simulink model "BLDC"  (R2023b)
settings: Solver=VariableStepAuto  StartTime=0.0  StopTime=0.25  RelTol=1e-3
libraries: simulink x6, spsPermanentMagnetSynchronousMachineLib x1, spsControlledVoltageSourceLib x1, slpidlib x1, spsUniversalBridgeLib x1, spsVoltageMeasurementLib x1, spspowerguiLib x1
settings Model: Creator=Akaashdeep B  LastModifiedBy=Akaashdeep B

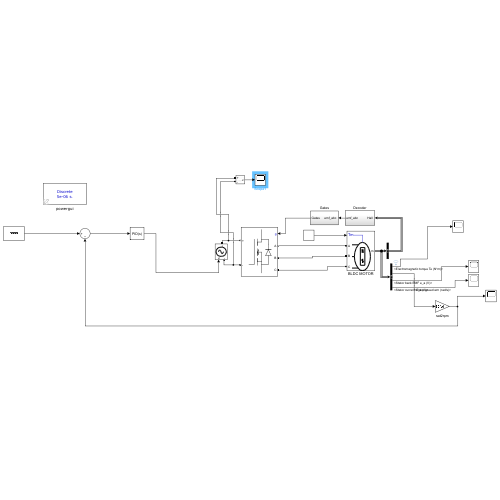
[thumbnail: Simulink's stored preview of the top-level diagram]
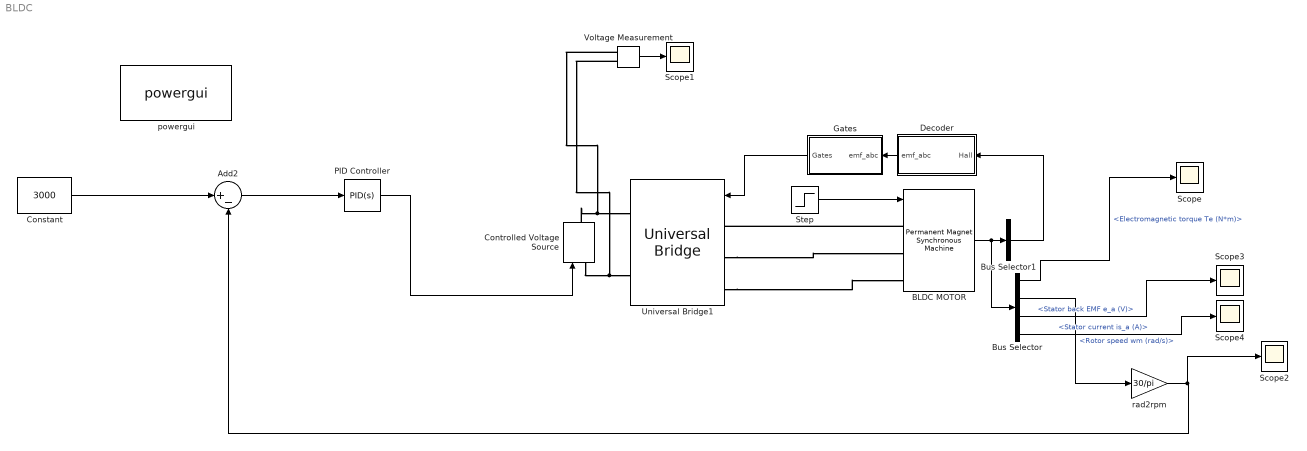
== system BLDC ==
  Add2 : Sum  Inputs=|+-
  BLDC MOTOR : spsPermanentMagnetSynchronousMachineLib/Permanent Magnet Synchronous Machine  NbPhases=3  FluxDistribution=Trapezoidal  RotorType=Round  MechanicalLoad=Torque Tm  PresetModel=No  ShowDetailedParameters=on  MeasurementBus=off  Resistance=2.8750  Inductance=8.5e-3  dqInductances=[8.5e-3, 8.5e-3]  La=0.000835  MachineConstant=Torque Constant (N.m / A_peak)  Flux=0.175  VoltageCst=146.6077  TorqueCst=1.4  Flat=120  Mechanical="[ 0.8e-3, 1e-3,  4 ]"  PolePairs=4  InitialConditions=[0,0, 0,0]  InitialConditions5ph=[0 0 0 0 0 0]  RefAngle=90 degrees behind phase A axis (modified Park)  IterativeDiscreteModel=Trapezoidal non iterative  TsBlock=-1  TsPowergui=0
  Bus Selector : BusSelector  OutputSignals=Electromagnetic torque Te (N*m),Rotor speed wm (rad/s),Stator back EMF e_a (V),Stator current is_a (A)
  Bus Selector1 : BusSelector  OutputSignals=Hall effect signal h_a,Hall effect signal h_b,Hall effect signal h_c  OutputAsBus=on
  Constant : Constant  Value=3000
  Controlled Voltage Source : spsControlledVoltageSourceLib/Controlled Voltage Source  Initialize=on  Source_Type=DC  Amplitude=0  Phase=0  Frequency=50  Measurements=None
  Decoder : Subsystem
  Gates : Subsystem
  PID Controller : slpidlib/PID Controller  Controller=PID  Form=Parallel  TimeDomain=Continuous-time  UseExternalTs=off  SampleTime=-1  IntegratorMethod=Forward Euler  FilterMethod=Forward Euler  ControllerParametersSource=internal  P=0.01035  I=12.777  UseKiTs=off  D=12.564  N=0  UseFilter=on  TunerSelectOption=Transfer Function Based (PID Tuner App)  InitialConditionSource=internal  InitialConditionForIntegrator=0  InitialConditionForFilter=0  DifferentiatorICPrevScaledInput=0  ExternalReset=none  TrackingMode=off  Kt=1  LimitOutput=off  SatLimitsSource=internal  UpperSaturationLimit=inf  LowerSaturationLimit=-inf  LinearizeAsGain=on  AntiWindupMode=none  Kb=1  LimitIntegrator=off  UpperIntegratorSaturationLimit=inf  LowerIntegratorSaturationLimit=-inf  POutMin=[]  POutMax=[]  IOutMin=[]  IOutMax=[]  DOutMin=[]  DOutMax=[]  NOutMin=[]  NOutMax=[]  SumOutMin=[]  SumOutMax=[]  SaturationOutMin=[]  SaturationOutMax=[]  PParamMin=[]  PParamMax=[]  IParamMin=[]  IParamMax=[]  DParamMin=[]  DParamMax=[]  NParamMin=[]  NParamMax=[]  KbParamMin=[]  KbParamMax=[]  KtParamMin=[]  KtParamMax=[]  KbOutMin=[]  KbOutMax=[]  KtOutMin=[]  KtOutMax=[]  IntegratorOutMin=[]  IntegratorOutMax=[]  FilterOutMin=[]  FilterOutMax=[]  SumI1OutMin=[]  SumI1OutMax=[]  SumI2OutMin=[]  SumI2OutMax=[]  SumI3OutMin=[]  SumI3OutMax=[]  SumI4OutMin=[]  SumI4OutMax=[]  SumDOutMin=[]  SumDOutMax=[]  DifferentiatorOutMin=[]  DifferentiatorOutMax=[]  FilterDiffOutCoefMin=[]  FilterDiffOutCoefMax=[]  ReciprocalOutMin=[]  ReciprocalOutMax=[]  SumDenOutMin=[]  SumDenOutMax=[]  SumNumOutMin=[]  SumNumOutMax=[]  DivideOutMin=[]  DivideOutMax=[]  UdiffTsProdOutMin=[]  UdiffTsProdOutMax=[]  NTsProdOutMin=[]  NTsProdOutMax=[]  UintegralTsProdOutMin=[]  UintegralTsProdOutMax=[]  UngainTsProdOutMin=[]  UngainTsProdOutMax=[]  ClampingZeroOutDataTypeStr=Inherit: Inherit via back propagation  ClampingZeroOutMin=[]  ClampingZeroOutMax=[]  FilterDenConstantOutDataTypeStr=Inherit: Inherit via back propagation  FilterDenConstantOutMin=[]  FilterDenConstantOutMax=[]  PCopyOutDataTypeStr=Inherit: Inherit via back propagation  PCopyOutMin=[]  PCopyOutMax=[]  NCopyOutDataTypeStr=Inherit: Inherit via back propagation  NCopyOutMin=[]  NCopyOutMax=[]  IntegratorContinuousStateAttributes=''  IntegratorStateMustResolveToSignalObject=off  IntegratorRTWStateStorageClass=Auto  FilterContinuousStateAttributes=''  FilterStateMustResolveToSignalObject=off  FilterRTWStateStorageClass=Auto  ParallelPVariant=InternalParameters  IdealPVariant=Disabled  IVariant=InternalParameters  DVariant=InternalParameters  IntegratorVariant=Continuous  SatVariant=Disabled  AWVariant=Passthrough  PCopyVariant=Disabled  TRVariant=Disabled  FdbkBlocksVariant=Forward  IdealPFdbkVariant=Disabled  SatFdbkVariant=Disabled  DerivativeFilterVariant=ContFilter  NVariant=InternalParameters  NCopyVariant=Disabled  FilterICVariant=InternalICsFilter  IntegratorICVariant=InternalICs  ExternalResetVariant=Disabled  TRSumVariant=Passthrough  SumFdbkVariant=Disabled  SumVariant=Sum_PID  TsampFilterVariant=InternalTs  TsampNgainVariant=Passthrough  TsampIntegralVariant=Disabled_SignalSpec  ExternalSaturationOutDataTypeStr=Inherit: Same as second input
  Scope{,1..4} (5 alike) : Scope
  Step : Step  Time=0.1  SampleTime=0
  Universal Bridge1 : spsUniversalBridgeLib/Universal Bridge  Arms=3  SnubberResistance=5000  SnubberCapacitance=1e-6  Device=MOSFET / Diodes  Ron=1e-3  Lon=0  ForwardVoltages="[  0  0  ]"  ForwardVoltage=0  GTOparameters=[ 10e-6 , 20e-6 ]  IGBTparameters=[ 1e-6 , 2e-6 ]  Measurements=None  Measurements_2=None  converterType=Rectifier
  Voltage Measurement : spsVoltageMeasurementLib/Voltage Measurement  PhasorSimulation=off  OutputType=Complex  PSBequivalent=0
  powergui : spspowerguiLib/powergui  SimulationMode=Discrete  SampleTime=5e-6  frequency=60  Iterations=50  frequencyindice=0  Pbase=100e6  ErrMax=1e-4  UnitsV=kV  UnitsW=MW  buscounter=0  FunctionMessages=off  echomessages=off  EnableUseOfTLC=off  CurrentSourceSwitches=off  DisableSnubberDevices=off  DisableRonSwitches=off  DisableVfSwitches=off  DisplayEquations=off  AutomaticDiscreteSolvers=off  SolverType=Tustin  Interpol=off  ExternalGateDelay=off  methode=off  Ts=0  x0status=blocks  SPID=off  SwTol=0  HookPort=off  NonlinearTolerance=1e-4  nMaxIteration=100  ContinueOnMaxIteration=off  RestoreLinks=warning  ResistiveCurrentMeasurement=off  Frange=[0:2:500]  Ylog=off  Xlog=on  ShowGrid=off  save=off  variable=ZData  structure=ScopeData7  ZoomFFT=off  StartTime=0.24  cycles=1  DisplayStyle=1  fundamental=50  FreqAxis=on  MaxFrequency=1000  frequencyindicesteady=1  RmsSteady=1  display=off
  rad2rpm : Gain  Gain=30/pi
  wires:
  PID Controller/1 -> Controlled Voltage Source/1
  Bus Selector/1 -> Scope/1  "<Electromagnetic torque Te (N*m)>"
  Gates/1(Gates) -> Universal Bridge1/1
  Bus Selector/2 -> rad2rpm/1  "<Rotor speed wm (rad/s)>"
  Decoder/1(emf_abc) -> Gates/1("emf_abc ")
  Bus Selector1/1 -> Decoder/1("Hall ")
  Add2/1 -> PID Controller/1
  Constant/1 -> Add2/1
  BLDC MOTOR/1 -> Bus Selector1/1, Bus Selector/1
  Step/1 -> BLDC MOTOR/1
  Voltage Measurement/1 -> Scope1/1
  rad2rpm/1 -> Scope2/1, Add2/2
  Bus Selector/3 -> Scope3/1  "<Stator back EMF e_a (V)>"
  Bus Selector/4 -> Scope4/1  "<Stator current is_a (A)>"
  connections:
  Universal Bridge1/LConn3 -- BLDC MOTOR/LConn3
  Universal Bridge1/LConn2 -- BLDC MOTOR/LConn2
  Controlled Voltage Source/RConn1 -- Voltage Measurement/LConn1 -- Universal Bridge1/RConn1
  BLDC MOTOR/LConn1 -- Universal Bridge1/LConn1
  Controlled Voltage Source/LConn1 -- Voltage Measurement/LConn2 -- Universal Bridge1/RConn2

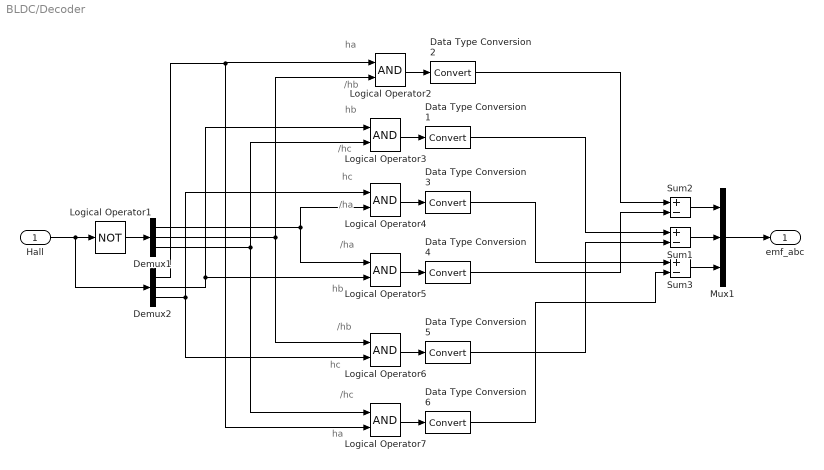
== system BLDC/Decoder ==
  note: ha
  note: /hc
  note: hc
  note: /hb
  note: hb
  note: /ha
  note: /ha
  note: hc
  note: /hc
  note: hb
  note: /hb
  note: ha
  "Hall " : Inport
  Data Type Conversion{1..6} (6 alike) : DataTypeConversion  SaturateOnIntegerOverflow=off  RndMeth=Floor
  Demux1 : Demux  Outputs=3
  Demux2 : Demux  Outputs=3
  Logical Operator1 : Logic  Operator=NOT  AllPortsSameDT=off  OutDataTypeStr=boolean
  Logical Operator{2..7} (6 alike) : Logic  AllPortsSameDT=off  OutDataTypeStr=boolean
  Mux1 : Mux  Inputs=3
  Sum1 : Sum  Inputs=+-  OutDataTypeStr=double
  Sum2 : Sum  Inputs=+-  OutDataTypeStr=double
  Sum3 : Sum  Inputs=+-  OutDataTypeStr=double
  emf_abc : Outport  VectorParamsAs1DForOutWhenUnconnected=off
  wires:
  Data Type Conversion6/1 -> Sum3/2
  Data Type Conversion3/1 -> Sum3/1
  Data Type Conversion5/1 -> Sum1/2
  Data Type Conversion1/1 -> Sum1/1
  Data Type Conversion4/1 -> Sum2/2
  Data Type Conversion2/1 -> Sum2/1
  Logical Operator7/1 -> Data Type Conversion6/1
  Logical Operator6/1 -> Data Type Conversion5/1
  Logical Operator5/1 -> Data Type Conversion4/1
  Logical Operator4/1 -> Data Type Conversion3/1
  Logical Operator3/1 -> Data Type Conversion1/1
  Mux1/1 -> emf_abc/1
  Sum3/1 -> Mux1/3
  Sum1/1 -> Mux1/2
  Sum2/1 -> Mux1/1
  Logical Operator2/1 -> Data Type Conversion2/1
  Demux1/1 -> Logical Operator5/1, Logical Operator4/2
  Demux1/2 -> Logical Operator6/1, Logical Operator2/2
  Demux1/3 -> Logical Operator7/1, Logical Operator3/2
  Demux2/1 -> Logical Operator7/2, Logical Operator2/1
  Demux2/2 -> Logical Operator5/2, Logical Operator3/1
  Demux2/3 -> Logical Operator6/2, Logical Operator4/1
  Logical Operator1/1 -> Demux1/1
  "Hall "/1 -> Demux2/1, Logical Operator1/1

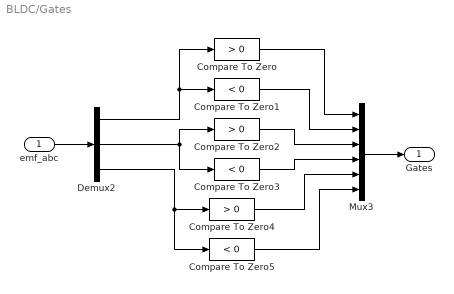
== system BLDC/Gates ==
  "emf_abc " : Inport
  Compare To Zero : simulink/Logic and Bit Operations/Compare To Zero  relop=>  OutDataTypeStr=boolean  ZeroCross=off
  Compare To Zero1 : simulink/Logic and Bit Operations/Compare To Zero  relop=<  OutDataTypeStr=boolean  ZeroCross=off
  Compare To Zero2 : simulink/Logic and Bit Operations/Compare To Zero  relop=>  OutDataTypeStr=boolean  ZeroCross=off
  Compare To Zero3 : simulink/Logic and Bit Operations/Compare To Zero  relop=<  OutDataTypeStr=boolean  ZeroCross=off
  Compare To Zero4 : simulink/Logic and Bit Operations/Compare To Zero  relop=>  OutDataTypeStr=boolean  ZeroCross=off
  Compare To Zero5 : simulink/Logic and Bit Operations/Compare To Zero  relop=<  OutDataTypeStr=boolean  ZeroCross=off
  Demux2 : Demux  Outputs=3
  Mux3 : Mux  Inputs=6
  Gates : Outport  VectorParamsAs1DForOutWhenUnconnected=off
  wires:
  Compare To Zero5/1 -> Mux3/6
  Compare To Zero4/1 -> Mux3/5
  Compare To Zero3/1 -> Mux3/4
  Compare To Zero2/1 -> Mux3/3
  Compare To Zero1/1 -> Mux3/2
  Compare To Zero/1 -> Mux3/1
  Demux2/3 -> Compare To Zero5/1, Compare To Zero4/1
  Demux2/2 -> Compare To Zero3/1, Compare To Zero2/1
  Demux2/1 -> Compare To Zero1/1, Compare To Zero/1
  Mux3/1 -> Gates/1
  "emf_abc "/1 -> Demux2/1
